simulink model "siude"  (Simulink 8.5)
settings: Solver=ode4  StartTime=0.0  StopTime=tstop  FixedStep=tstep  RelTol=1e-3
values from neighbouring files (symbols this model uses):
  bnom = Kq*(Mn^2)*dm*wa    (= -3680.56065687)    [dataude.m]
  tau = 0.01    [dataude.m]
settings Model: Creator=Dr SE Talole  LastModifiedBy=Vish
settings OptimizationCC: InitFltsAndDblsToZero=on
settings DebuggingCC: SaveWithParameterizedLinksMsg=none  SignalResolutionControl=TryResolveAllWithWarning  SolverPrmCheckMsg=warning  MultiTaskDSMMsg=warning  MultiTaskCondExecSysMsg=none  FcnCallInpInsideContextMsg=UseLocalSettings
settings GRTTargetCC: TargetFcnLib=ansi_tfl_tmw.mat

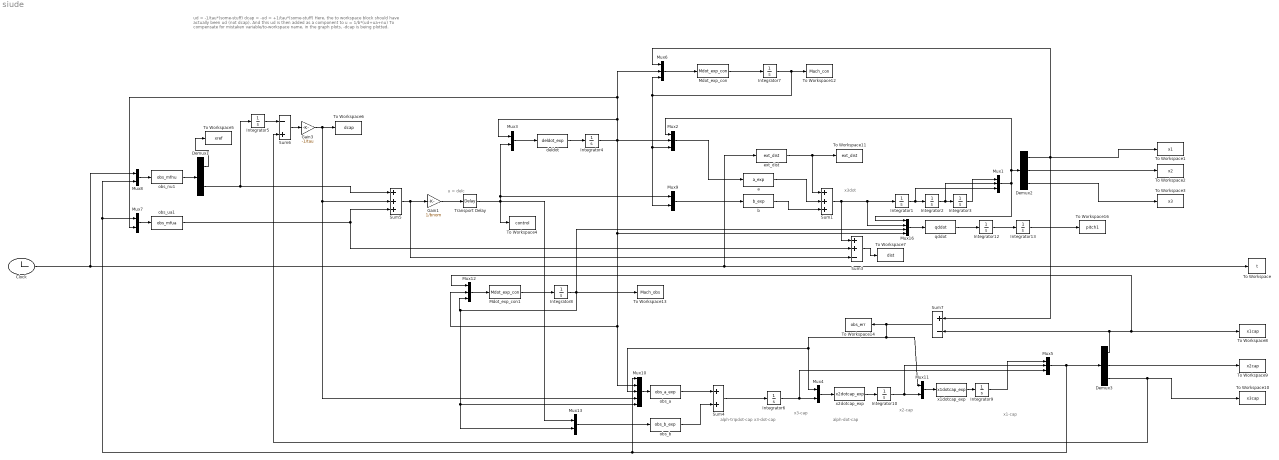
== system siude ==
  note: ud = -1/tau*(some-stuff)
      | dcap = -ud = +1/tau*(some-stuff)
      | Here, the to workspace block should have actually been ud (not dcap).
      | And this ud is then added as a component to u = 1/b*(ud+ua+nu)
      |
      | To compensate for mistaken variable/to-workspace name, in the graph
      | plots, -dcap is being plotted.
  note: x2-cap
  note: alph-tripdot-cap
      | x3-dot-cap
  note: u = delc
  note: x3dot
  note: x3-cap
  note: alph-dot-cap
  note: x1-cap
  Clock : Clock
  Demux1 : Demux  Outputs=2
  Demux2 : Demux  Outputs=3
  Demux3 : Demux  Outputs=3
  Gain1 : Gain  Gain=1/bnom
  Gain3 : Gain  Gain=-1/tau
  Integrator{1..6,9..10,12..13} (10 alike) : Integrator
  Integrator7 : Integrator  InitialCondition=2.5
  Integrator8 : Integrator  InitialCondition=2.5
  Mdot_exp_con : MATLABFcn  MATLABFcn=Mdot_exp_con  OutputDimensions=1
  Mdot_exp_con1 : MATLABFcn  MATLABFcn=Mdot_exp_con  OutputDimensions=1
  Mux{1..2,5..6,12} (5 alike) : Mux  Inputs=3
  Mux10 : Mux  Inputs=5
  Mux{3..4,7..9,11,13} (7 alike) : Mux  Inputs=2
  Mux16 : Mux
  Sum1 : Sum  Inputs=+++
  Sum3 : Sum  Inputs=++-
  Sum4 : Sum
  Sum5 : Sum  Inputs=+++
  Sum6 : Sum  Inputs=-+
  Sum7 : Sum  Inputs=+-
  To Workspace : ToWorkspace  VariableName=t  SampleTime=-1
  To Workspace1 : ToWorkspace  VariableName=x1  SampleTime=-1
  To Workspace10 : ToWorkspace  VariableName=x3cap  SampleTime=-1
  To Workspace11 : ToWorkspace  VariableName=ext_dist  SampleTime=-1
  To Workspace12 : ToWorkspace  VariableName=Mach_con  SampleTime=-1
  To Workspace13 : ToWorkspace  VariableName=Mach_obs  SampleTime=-1
  To Workspace14 : ToWorkspace  VariableName=obs_err  SampleTime=-1
  To Workspace16 : ToWorkspace  VariableName=pitch1  SampleTime=-1
  To Workspace2 : ToWorkspace  VariableName=x2  SampleTime=-1
  To Workspace3 : ToWorkspace  VariableName=x3  SampleTime=-1
  To Workspace4 : ToWorkspace  VariableName=control  SampleTime=-1
  To Workspace5 : ToWorkspace  VariableName=xref  SampleTime=-1
  To Workspace6 : ToWorkspace  VariableName=dcap  SampleTime=-1
  To Workspace7 : ToWorkspace  VariableName=dist  SampleTime=-1
  To Workspace8 : ToWorkspace  VariableName=x1cap  SampleTime=-1
  To Workspace9 : ToWorkspace  VariableName=x2cap  SampleTime=-1
  Transport Delay : TransportDelay  DelayTime=0.001
  a : MATLABFcn  MATLABFcn=a_exp  OutputDimensions=1
  b : MATLABFcn  MATLABFcn=b_exp  OutputDimensions=1
  deldot : MATLABFcn  MATLABFcn=deldot_exp  OutputDimensions=1
  ext_dist : MATLABFcn  MATLABFcn=ext_dist  OutputDimensions=1
  obs_a : MATLABFcn  MATLABFcn=obs_a_exp  OutputDimensions=1
  obs_b : MATLABFcn  MATLABFcn=obs_b_exp  OutputDimensions=1
  obs_nu1 : MATLABFcn  MATLABFcn=obs_mfnu  OutputDimensions=2
  obs_ua1 : MATLABFcn  MATLABFcn=obs_mfua  OutputDimensions=1
  qddot : MATLABFcn  MATLABFcn=qddot  OutputDimensions=1
  x1dotcap_exp : MATLABFcn  MATLABFcn=x1dotcap_exp  OutputDimensions=1
  x2dotcap_exp : MATLABFcn  MATLABFcn=x2dotcap_exp  OutputDimensions=1
  wires:
  Integrator3/1 -> Mux1/1
  Integrator2/1 -> Mux1/2, Integrator3/1
  Integrator1/1 -> Mux1/3, Integrator2/1
  Demux2/2 -> To Workspace2/1
  a/1 -> Sum1/2
  Mux2/1 -> a/1
  Demux2/3 -> To Workspace3/1
  Sum1/1 -> Mux16/2, Integrator1/1, Sum3/1
  Mux1/1 -> Mux16/1, Mux2/1, Demux2/1
  Gain1/1 -> Transport Delay/1
  Clock/1 -> To Workspace/1, ext_dist/1, Mux8/1
  Integrator9/1 -> Mux5/1
  Integrator10/1 -> Mux11/2, Mux5/2
  obs_b/1 -> Sum4/2
  Sum4/1 -> Integrator6/1
  obs_a/1 -> Sum4/1
  Demux3/2 -> To Workspace9/1
  Demux3/1 -> Sum7/2, Mux12/1, To Workspace8/1
  Mux8/1 -> obs_nu1/1
  Mux7/1 -> obs_ua1/1
  obs_nu1/1 -> Demux1/1
  Demux1/1 -> To Workspace5/1
  Demux1/2 -> Integrator5/1, Sum5/1
  obs_ua1/1 -> Sum3/2, Sum5/3
  Integrator5/1 -> Sum6/1
  Sum6/1 -> Gain3/1
  Gain3/1 -> To Workspace6/1, Mux10/4, Sum5/2
  Demux3/3 -> Sum6/2, To Workspace10/1
  Sum5/1 -> Sum3/3, Gain1/1
  deldot/1 -> Integrator4/1
  Mux3/1 -> deldot/1
  Sum3/1 -> To Workspace7/1
  b/1 -> Sum1/3
  Mux10/1 -> obs_a/1
  Sum7/1 -> To Workspace14/1, Mux11/1, Mux4/1, Mux10/3
  Integrator6/1 -> Mux5/3, Mux4/2
  x2dotcap_exp/1 -> Integrator10/1
  x1dotcap_exp/1 -> Integrator9/1
  Mux5/1 -> Mux8/2, Mux7/1, Mux10/1, Demux3/1
  Mux4/1 -> x2dotcap_exp/1
  Mux11/1 -> x1dotcap_exp/1
  ext_dist/1 -> Sum1/1, To Workspace11/1
  Mux6/1 -> Mdot_exp_con/1
  Mdot_exp_con/1 -> Integrator7/1
  Integrator7/1 -> To Workspace12/1, Mux6/3, Mux9/2, Mux2/3
  Demux2/1 -> Mux6/1, Sum7/1, To Workspace1/1
  Mux9/1 -> b/1
  Mdot_exp_con1/1 -> Integrator8/1
  Mux12/1 -> Mdot_exp_con1/1
  Integrator8/1 -> Mux16/3, Mux13/2, Mux10/5, Mux12/3, To Workspace13/1
  Mux13/1 -> obs_b/1
  Mux16/1 -> qddot/1
  qddot/1 -> Integrator12/1
  Integrator12/1 -> Integrator13/1
  Integrator13/1 -> To Workspace16/1
  Integrator4/1 -> Mux10/2, Mux12/2, Mux16/4, Mux7/2, Mux6/2, Mux3/1, Mux2/2
  Transport Delay/1 -> Mux13/1, Mux3/2, Mux9/1, To Workspace4/1
